simulink model "sampleModel1868"  (R2023a)
settings: Solver=VariableStepAuto  StartTime=0.0  StopTime=10.0  RelTol=1e-3
libraries: simulink x6, hdlsllib x3
settings Model: Creator=user1  LastModifiedBy=user1

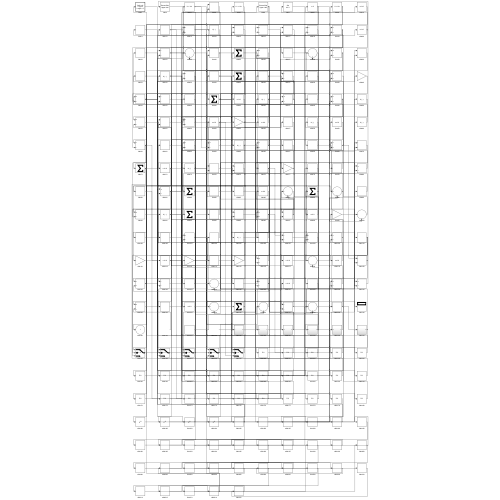
[thumbnail: Simulink's stored preview of the top-level diagram]
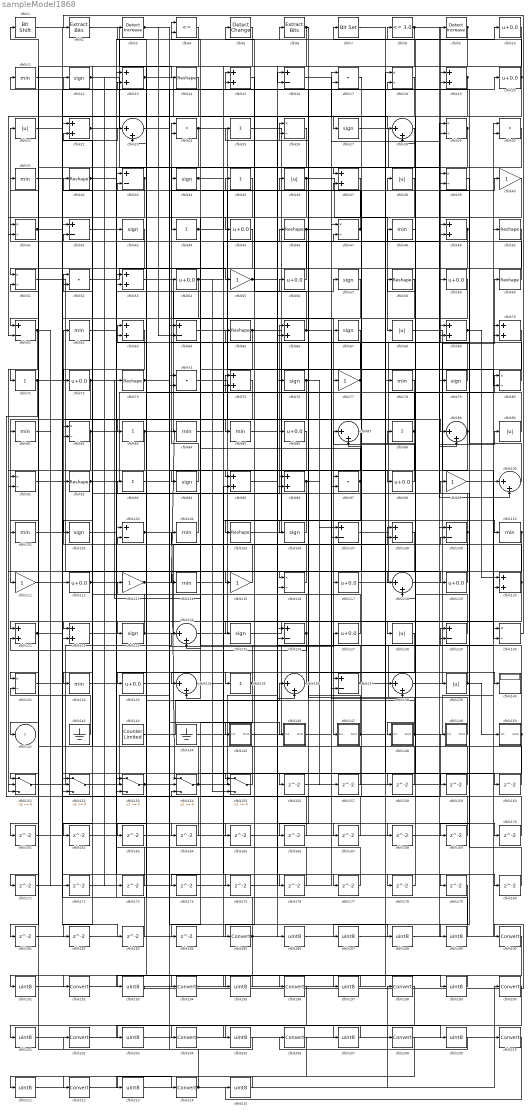
== system sampleModel1868 ==
  cfblk1 : hdlsllib/Logic and Bit Operations/Bit Shift  mode=Shift Left Logical  N=0
  cfblk{10,20,45,54,56,59,72,86,98,112,117,119,127,133} (14 alike) : Bias  Bias=0.0  SaturateOnIntegerOverflow=off
  cfblk{23,28,87,89,100,118,124,134,136,138} (10 alike) : Sum  Inputs=|++
  cfblk{11,31,48,62,78,81,84..85,101,104,110,114,132} (13 alike) : MinMax
  cfblk{12,27,34,43,57,67,76,79,94,102,106,123,125} (13 alike) : Signum
  cfblk{16,33,42,61,64,103,107,109,126,129,137} (11 alike) : Sum  Inputs=+-
  cfblk{14,32,46,50,58,60,65,73,92,105} (10 alike) : Reshape
  cfblk{13,15,19,22,37,49,53,63,66,69..70,75,95..96,108,120..122} (18 alike) : Sum
  cfblk{40,55,77,99,111,113,115} (7 alike) : Gain
  cfblk{18,26,29,39,41,47,51,80,82,91,116,130..131} (13 alike) : Product  Inputs=*/  RndMeth=Zero  SaturateOnIntegerOverflow=on
  cfblk{21,36,38,68,90,128,139} (7 alike) : Abs  SaturateOnIntegerOverflow=off
  cfblk{25,35,44,71,83,88,93,135} (8 alike) : Sum  Inputs=+
  cfblk140 : Display
  cfblk142 : Ground
  cfblk143 : hdlsllib/Sources/Counter Limited  uplimit=7  tsamp=-1
  cfblk144 : Ground
  cfblk145 : Subsystem
      settings: LibrarySourceBlock=|
      | hdlsllib/Ports &
      | Subsystems/Subsystem
  cfblk146 : Subsystem
      settings: LibrarySourceBlock=|
      | hdlsllib/Ports &
      | Subsystems/Subsystem
  cfblk147 : Subsystem
      settings: LibrarySourceBlock=|
      | hdlsllib/Ports &
      | Subsystems/Subsystem
  cfblk148 : Subsystem
      settings: LibrarySourceBlock=|
      | hdlsllib/Ports &
      | Subsystems/Subsystem
  cfblk149 : Subsystem
      settings: LibrarySourceBlock=|
      | hdlsllib/Ports &
      | Subsystems/Subsystem
  cfblk150 : Subsystem
      settings: LibrarySourceBlock=|
      | hdlsllib/Ports &
      | Subsystems/Subsystem
  cfblk{151..155} (5 alike) : Switch  SaturateOnIntegerOverflow=off  InputSameDT=off
  cfblk{156..184} (29 alike) : Delay  SampleTime=1
  cfblk{17,24,30,52,74,97} (6 alike) : DotProduct  OutDataTypeStr=Inherit: Inherit via internal rule
  cfblk{185,190,192,194,196,198,200,202,204,206,208,210,212,214} (14 alike) : DataTypeConversion  SaturateOnIntegerOverflow=off  RndMeth=Floor
  cfblk{186..189,191,193,195,197,199,201,203,205,207,209,211,213,215} (17 alike) : DataTypeConversion  OutDataTypeStr=uint8  SaturateOnIntegerOverflow=off  RndMeth=Floor
  cfblk2 : simulink/Logic and Bit Operations/Extract Bits  bitsToExtract=Upper half  numBits=8  bitIdxRange=[0 7]  outScalingMode=Preserve fixed-point scaling
      settings: LibrarySourceBlock=|
      | hdlsllib/Logic and Bit
      | Operations/Extract Bits
  cfblk3 : simulink/Logic and Bit Operations/Detect Increase  vinit=0.0  OutDataTypeStr=boolean
      settings: LibrarySourceBlock=|
      | hdlsllib/Logic and Bit
      | Operations/Detect
      | Increase
  cfblk4 : RelationalOperator  Operator=<=  OutDataTypeStr=boolean  InputSameDT=off
  cfblk5 : simulink/Logic and Bit Operations/Detect Change  vinit=0  OutDataTypeStr=boolean
      settings: LibrarySourceBlock=|
      | hdlsllib/Logic and Bit
      | Operations/Detect
      | Change
  cfblk6 : simulink/Logic and Bit Operations/Extract Bits  bitsToExtract=Upper half  numBits=8  bitIdxRange=[0 7]  outScalingMode=Preserve fixed-point scaling
      settings: LibrarySourceBlock=|
      | hdlsllib/Logic and Bit
      | Operations/Extract Bits
  cfblk7 : simulink/Logic and Bit Operations/Bit Set  iBit=0
      settings: LibrarySourceBlock=|
      | hdlsllib/Logic and Bit
      | Operations/Bit Set
  cfblk8 : hdlsllib/Logic and Bit Operations/Compare To Constant  relop=<=  const=3.0  OutDataTypeStr=boolean
  cfblk9 : simulink/Logic and Bit Operations/Detect Increase  vinit=0.0  OutDataTypeStr=boolean
      settings: LibrarySourceBlock=|
      | hdlsllib/Logic and Bit
      | Operations/Detect
      | Increase
  cfblk141 : Outport  VectorParamsAs1DForOutWhenUnconnected=off
  wires:
  cfblk59/1 -> cfblk147/1(In1)
  cfblk107/1 -> cfblk12/1
  cfblk50/1 -> cfblk51/1
  cfblk138/1 -> cfblk60/1
  cfblk127/1 -> cfblk113/1
  cfblk125/1 -> cfblk128/1
  cfblk136/1 -> cfblk73/1
  cfblk117/1 -> cfblk80/1
  cfblk83/1 -> cfblk57/1, cfblk152/3
  cfblk109/1 -> cfblk118/1, cfblk52/2
  cfblk72/1 -> cfblk111/1, cfblk176/1
  cfblk123/1 -> cfblk108/1, cfblk52/1
  cfblk94/1 -> cfblk24/1
  cfblk81/1 -> cfblk112/1
  cfblk51/1 -> cfblk119/1
  cfblk130/1 -> cfblk2/1
  cfblk149/1(Out1) -> cfblk118/2
  cfblk25/1 -> cfblk110/1
  cfblk49/1 -> cfblk123/1, cfblk96/2
  cfblk86/1 -> cfblk133/1
  cfblk22/1 -> cfblk10/1, cfblk69/2
  cfblk99/1 -> cfblk70/1
  cfblk124/1 -> cfblk38/1
  cfblk106/1 -> cfblk66/1
  cfblk34/1 -> cfblk177/1, cfblk178/1
  cfblk150/1(Out1) -> cfblk88/1, cfblk184/1
  cfblk6/1 -> cfblk116/1, cfblk75/2
  cfblk118/1 -> cfblk90/1
  cfblk113/1 -> cfblk84/1, cfblk137/1
  cfblk80/1 -> cfblk9/1
  cfblk5/1 -> cfblk71/1
  cfblk24/1 -> cfblk80/2, cfblk53/2
  cfblk103/1 -> cfblk154/1, cfblk146/1(In1)
  cfblk11/1 -> cfblk27/1
  cfblk102/1 -> cfblk43/1
  cfblk48/1 -> cfblk8/1
  cfblk52/1 -> cfblk55/1
  cfblk30/1 -> cfblk185/1
  cfblk35/1 -> cfblk134/1
  cfblk92/1 -> cfblk17/1, cfblk164/1
  cfblk28/1 -> cfblk95/1
  cfblk54/1 -> cfblk122/1, cfblk47/2, cfblk155/3
  cfblk70/1 -> cfblk134/2
  cfblk105/1 -> cfblk59/1
  cfblk119/1 -> cfblk62/1
  cfblk40/1 -> cfblk61/1
  cfblk13/1 -> cfblk76/1, cfblk98/1
  cfblk129/1 -> cfblk87/1
  cfblk120/1 -> cfblk99/1, cfblk171/1
  cfblk68/1 -> cfblk130/1
  cfblk18/1 -> cfblk115/1
  cfblk37/1 -> cfblk94/1
  cfblk45/1 -> cfblk74/2
  cfblk53/1 -> cfblk67/1
  cfblk61/1 -> cfblk151/2, cfblk172/1
  cfblk20/1 -> cfblk7/1, cfblk158/1
  cfblk21/1 -> cfblk85/1
  cfblk153/1 -> cfblk127/1, cfblk13/2
  cfblk4/1 -> cfblk121/1
  cfblk151/1 -> cfblk124/1
  cfblk104/1 -> cfblk32/1
  cfblk77/1 -> cfblk24/2, cfblk91/1
  cfblk47/1 -> cfblk4/1, cfblk97/1
  cfblk133/1 -> cfblk135/1
  cfblk114/1 -> cfblk130/2
  cfblk115/1 -> cfblk103/2
  cfblk122/1 -> cfblk4/2
  cfblk147/1(Out1) -> cfblk25/1, cfblk19/2, cfblk15/1
  cfblk116/1 -> cfblk92/1
  cfblk108/1 -> cfblk126/2
  cfblk112/1 -> cfblk65/1, cfblk165/1
  cfblk33/1 -> cfblk102/1, cfblk141/1
  cfblk148/1(Out1) -> cfblk100/1, cfblk75/1, cfblk23/2
  cfblk29/1 -> cfblk44/1, cfblk161/1
  cfblk137/1 -> cfblk70/2, cfblk26/2
  cfblk145/1(Out1) -> cfblk50/1
  cfblk58/1 -> cfblk132/1
  cfblk64/1 -> cfblk17/2
  cfblk143/1 -> cfblk136/1
  cfblk110/1 -> cfblk151/3, cfblk120/2, cfblk189/1
  cfblk132/1 -> cfblk96/1
  cfblk76/1 -> cfblk131/1, cfblk107/1
  cfblk131/1 -> cfblk40/1
  cfblk66/1 -> cfblk5/1, cfblk138/2
  cfblk101/1 -> cfblk114/1
  cfblk126/1 -> cfblk42/2, cfblk121/2
  cfblk135/1 -> cfblk104/1, cfblk174/1
  cfblk56/1 -> cfblk21/1
  cfblk2/1 -> cfblk14/1
  cfblk65/1 -> cfblk124/2, cfblk77/1
  cfblk139/1 -> cfblk11/1, cfblk150/1(In1)
  cfblk19/1 -> cfblk148/1(In1), cfblk61/2, cfblk181/1
  cfblk152/1 -> cfblk56/1
  cfblk154/1 -> cfblk129/1, cfblk3/1
  cfblk12/1 -> cfblk37/1, cfblk173/1
  cfblk87/1 -> cfblk106/1
  cfblk8/1 -> cfblk100/2, cfblk155/2, cfblk182/1
  cfblk155/1 -> cfblk63/1
  cfblk95/1 -> cfblk49/1
  cfblk41/1 -> cfblk33/2, cfblk153/2, cfblk23/1
  cfblk17/1 -> cfblk117/1
  cfblk42/1 -> cfblk89/1
  cfblk27/1 -> cfblk79/1
  cfblk32/1 -> cfblk153/1, cfblk137/2
  cfblk97/1 -> cfblk86/1, cfblk155/1, cfblk34/1
  cfblk71/1 -> cfblk149/1(In1), cfblk15/2
  cfblk9/1 -> cfblk101/1, cfblk163/1
  cfblk60/1 -> cfblk46/1
  cfblk15/1 -> cfblk45/1
  cfblk44/1 -> cfblk36/1, cfblk107/2, cfblk140/1
  cfblk36/1 -> cfblk68/1, cfblk41/2
  cfblk84/1 -> cfblk69/1
  cfblk79/1 -> cfblk37/2
  cfblk63/1 -> cfblk72/1
  cfblk98/1 -> cfblk35/1
  cfblk142/1 -> cfblk131/2
  cfblk121/1 -> cfblk51/2, cfblk168/1
  cfblk144/1 -> cfblk39/1
  cfblk67/1 -> cfblk116/2
  cfblk96/1 -> cfblk125/1, cfblk157/1
  cfblk1/1 -> cfblk83/1
  cfblk43/1 -> cfblk82/2
  cfblk3/1 -> cfblk64/2, cfblk180/1
  cfblk73/1 -> cfblk20/1, cfblk145/1(In1)
  cfblk74/1 -> cfblk136/2
  cfblk16/1 -> cfblk28/1
  cfblk82/1 -> cfblk6/1, cfblk151/1, cfblk54/1
  cfblk26/1 -> cfblk122/2
  cfblk146/1(Out1) -> cfblk19/1
  cfblk89/1 -> cfblk105/1, cfblk26/1
  cfblk46/1 -> cfblk29/2, cfblk153/3
  cfblk10/1 -> cfblk16/2
  cfblk90/1 -> cfblk58/1
  cfblk88/1 -> cfblk63/2, cfblk91/2
  cfblk55/1 -> cfblk18/2, cfblk48/1
  cfblk75/1 -> cfblk81/1
  cfblk57/1 -> cfblk152/2
  cfblk100/1 -> cfblk41/1
  cfblk69/1 -> cfblk39/2, cfblk120/1
  cfblk128/1 -> cfblk156/1
  cfblk156/1 -> cfblk89/2
  cfblk157/1 -> cfblk1/1
  cfblk158/1 -> cfblk22/2
  cfblk7/1 -> cfblk159/1
  cfblk159/1 -> cfblk42/1
  cfblk62/1 -> cfblk160/1
  cfblk160/1 -> cfblk74/1
  cfblk161/1 -> cfblk18/1
  cfblk14/1 -> cfblk162/1
  cfblk162/1 -> cfblk108/2
  cfblk163/1 -> cfblk138/1
  cfblk164/1 -> cfblk154/3
  cfblk165/1 -> cfblk29/1
  cfblk38/1 -> cfblk166/1
  cfblk166/1 -> cfblk82/1
  cfblk91/1 -> cfblk167/1
  cfblk167/1 -> cfblk126/1
  cfblk168/1 -> cfblk129/2
  cfblk39/1 -> cfblk169/1
  cfblk169/1 -> cfblk87/2
  cfblk134/1 -> cfblk170/1
  cfblk170/1 -> cfblk16/1
  cfblk171/1 -> cfblk66/2
  cfblk172/1 -> cfblk33/1
  cfblk173/1 -> cfblk13/1
  cfblk174/1 -> cfblk97/2
  cfblk111/1 -> cfblk175/1
  cfblk175/1 -> cfblk47/1
  cfblk176/1 -> cfblk154/2
  cfblk177/1 -> cfblk103/1
  cfblk178/1 -> cfblk28/2
  cfblk23/1 -> cfblk179/1
  cfblk180/1 -> cfblk109/2
  cfblk181/1 -> cfblk95/2
  cfblk182/1 -> cfblk49/2
  cfblk31/1 -> cfblk183/1
  cfblk183/1 -> cfblk152/1
  cfblk184/1 -> cfblk139/1
  cfblk185/1 -> cfblk53/1, cfblk22/1, cfblk191/1
  cfblk85/1 -> cfblk186/1
  cfblk186/1 -> cfblk30/1
  cfblk179/1 -> cfblk187/1
  cfblk187/1 -> cfblk30/2
  cfblk93/1 -> cfblk188/1
  cfblk188/1 -> cfblk109/1
  cfblk189/1 -> cfblk93/1
  cfblk191/1 -> cfblk78/1
  cfblk78/1 -> cfblk193/1
  cfblk193/1 -> cfblk190/1
  cfblk190/1 -> cfblk195/1
  cfblk195/1 -> cfblk192/1
  cfblk192/1 -> cfblk197/1
  cfblk197/1 -> cfblk194/1
  cfblk194/1 -> cfblk199/1
  cfblk199/1 -> cfblk196/1
  cfblk196/1 -> cfblk201/1
  cfblk201/1 -> cfblk198/1
  cfblk198/1 -> cfblk203/1
  cfblk203/1 -> cfblk200/1
  cfblk200/1 -> cfblk205/1
  cfblk205/1 -> cfblk202/1
  cfblk202/1 -> cfblk207/1
  cfblk207/1 -> cfblk204/1
  cfblk204/1 -> cfblk209/1
  cfblk209/1 -> cfblk206/1
  cfblk206/1 -> cfblk211/1
  cfblk211/1 -> cfblk208/1
  cfblk212/1 -> cfblk214/1
  cfblk208/1 -> cfblk213/1
  cfblk213/1 -> cfblk210/1
  cfblk214/1 -> cfblk31/1, cfblk64/1
  cfblk210/1 -> cfblk215/1
  cfblk215/1 -> cfblk212/1

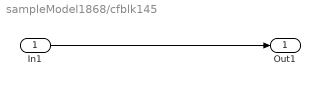
== system sampleModel1868/cfblk145 ==
  In1 : Inport
  Out1 : Outport
  wires:
  In1/1 -> Out1/1

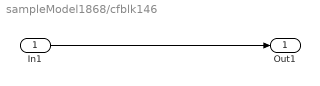
== system sampleModel1868/cfblk146 ==
  In1 : Inport
  Out1 : Outport
  wires:
  In1/1 -> Out1/1

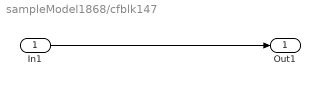
== system sampleModel1868/cfblk147 ==
  In1 : Inport
  Out1 : Outport
  wires:
  In1/1 -> Out1/1

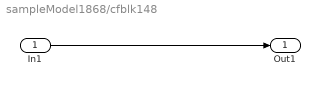
== system sampleModel1868/cfblk148 ==
  In1 : Inport
  Out1 : Outport
  wires:
  In1/1 -> Out1/1

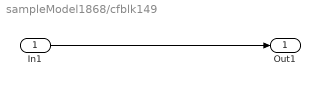
== system sampleModel1868/cfblk149 ==
  In1 : Inport
  Out1 : Outport
  wires:
  In1/1 -> Out1/1

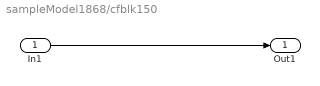
== system sampleModel1868/cfblk150 ==
  In1 : Inport
  Out1 : Outport
  wires:
  In1/1 -> Out1/1
